simulink model "fb_inverter_pwm2"  (Simulink 6.1)
settings: Solver=ode23tb  StartTime=0.0  StopTime=0.0599  MaxStep=1e-5  RelTol=1e-3  AbsTol=.01
libraries: powerlib x7, simulink x1
settings Model: LastModifiedBy=ThinkPad
settings DebuggingCC: SolverPrmCheckMsg=warning

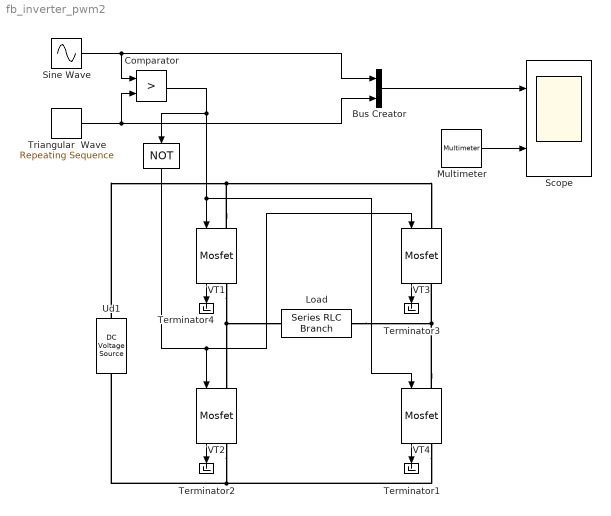
== system fb_inverter_pwm2 ==
  " " : Logic  Orientation=down  Operator=NOT  AllPortsSameDT=off  OutDataTypeMode=Boolean
  Bus Creator : BusCreator  DialogController=Simulink.DDGSource_Bus  Inputs=2
  Comparator : RelationalOperator  Operator=>  LogicOutDataTypeMode=Boolean  LogicDataType=sint(32)
  Load : powerlib/Elements/Series RLC Branch  PhysicalDomain=powersysdomain  SubClassName=unknown  LeftPortType=p1  RightPortType=p1  LConnTagsString=__new0  RConnTagsString=__new0  Resistance=1  Inductance=0.01  Capacitance=inf  Measurements=Branch voltage and current
  Multimeter : powerlib/Measurements/Multimeter  PhasorSimulation=off  OutputType=Complex  sel=[1 2]  L=2  Gain=[1 1]  yselected={'Ub: Load','Ib: Load'};  PSBOutputType=1  PSBequivalent=0  AxesSetting=[0,0.1,-100,100]  Display=0  SavedBlockNames=-11
  Scope : Scope  NumInputPorts=2
      settings: TimeRange=0.03  YMin=-1.5~-150  YMax=1.5~150  SampleTime=2e-4
  Sine Wave : Sin  Amplitude=0.8  Frequency=314  SampleTime=0
  Terminator{1..4} (4 alike) : Terminator
      settings: Orientation=down
  Triangular  Wave : simulink/Sources/Repeating Sequence  rep_seq_t=[0 2.5e-4 5e-4 7.5e-4 1e-3]  rep_seq_y=[0 1 0 -1 0]
  Ud1 : powerlib/Electrical Sources/DC Voltage Source  Orientation=up  Amplitude=100  Measurements=None
  VT{1..4} (4 alike) : powerlib/Power Electronics/Mosfet  Orientation=down  Ron=0.01  Lon=1e-7  Rd=.01  IC=0  Rs=5  Cs=1e-6  Measurements=on
  wires:
  Comparator/1 -> " "/1, VT1/1, VT4/1
  VT4/1 -> Terminator1/1
  VT2/1 -> Terminator2/1
  VT3/1 -> Terminator3/1
  Sine Wave/1 -> Comparator/1, Bus Creator/1
  Triangular  Wave/1 -> Comparator/2, Bus Creator/2
  Bus Creator/1 -> Scope/1
  " "/1 -> VT2/1, VT3/1
  Multimeter/1 -> Scope/2
  VT1/1 -> Terminator4/1
  connections:
  VT4/LConn1 -- VT3/RConn1 -- Load/RConn1
  VT1/RConn1 -- VT2/LConn1 -- Load/LConn1
  VT4/RConn1 -- Ud1/LConn1 -- VT2/RConn1
  VT1/LConn1 -- VT3/LConn1 -- Ud1/RConn1
